simulink model "SRS_MBC_Ioniq5_17_Carsim_ACC_final"  (R2023b)
settings: Solver=FixedStepAuto  StartTime=0.0  StopTime=200  FixedStep=0.001  MaxStep=0.001  RelTol=1e-3
libraries: slpidlib x3, Solver_SF x1
settings Model: DataTypeOverride=Double  MinMaxOverflowLogging=ForceOff  PacingRate=1.100000  Creator=황수빈  LastModifiedBy=황수빈

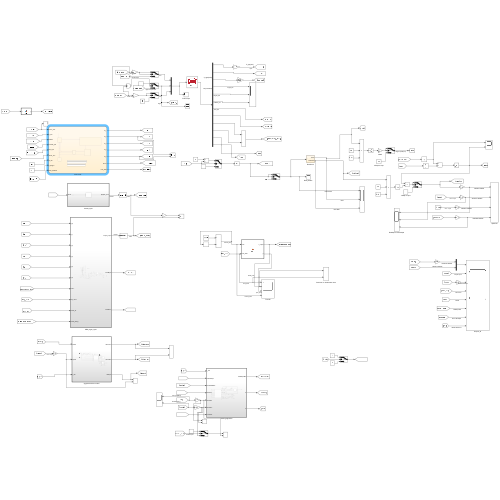
[thumbnail: Simulink's stored preview of the top-level diagram]
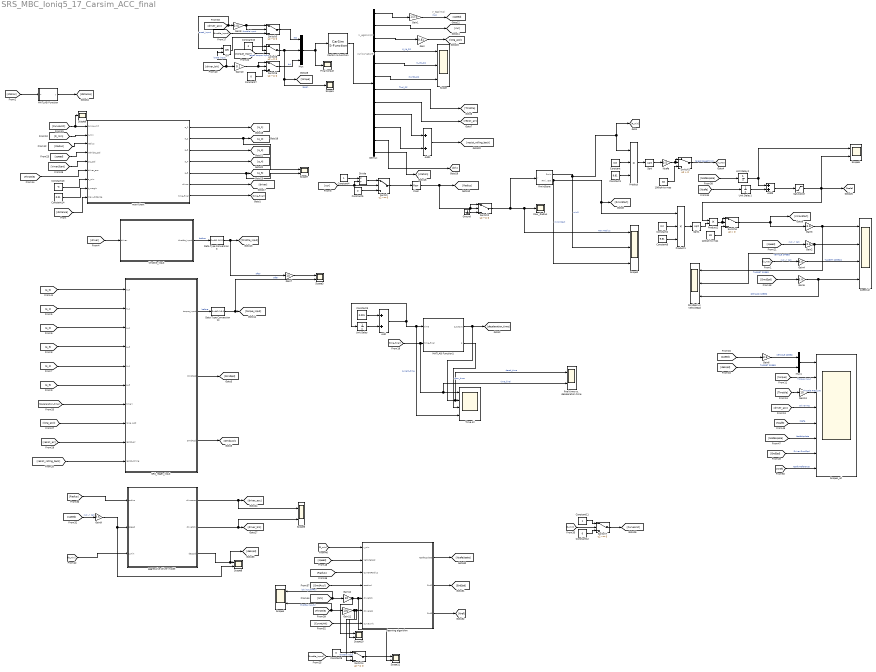
== system SRS_MBC_Ioniq5_17_Carsim_ACC_final ==
  note: V_ego(km/h)
  note: V_ego(m/s)
  note: cur(curvature)
  100kph to mps : Constant  Value=33
  120kph to mps : Constant  Value=33
  Add : Sum
  Add1 : Sum
  Add3 : Sum
  CarSim S-Function : Solver_SF/CarSim S-Function  Priority=1  SIMFILE=simfile.sim  Run_RTs=off  vs_state_ind=Run  StopMode_ind=Vehicle Model
  Constant : Constant  Value=0.8
  Constant1 : Constant  Value=9.81
  Constant{5,7..8,10,12} (5 alike) : Constant  Value=0
  Constant11 : Constant
  Constant13 : Constant  Value=-3
  Constant14 : Constant  Value=0.01
  Constant2 : Constant  Value=0.2
  Constant3 : Constant  Value=0.001
  Constant4 : Constant
  Constant6 : Constant  Value=9.81
  Data Type Conversion14 : DataTypeConversion  OutDataTypeStr=fixdt(1,16,0)  RndMeth=Nearest  SaturateOnIntegerOverflow=off
  Data Type Conversion3 : DataTypeConversion  OutDataTypeStr=fixdt(1,16,0)  RndMeth=Nearest  SaturateOnIntegerOverflow=off
  Demux : Demux  Outputs=12
  Divide : Product  Inputs=*/
  DmdSpd vs VehicleSpd : Scope  NumInputPorts=3
  Final torque : Scope
  Floor : Rounding
  Gain : Gain  Gain=9.81
  Gain1 : Gain  Gain=1/3.6
  Gain10 : Gain  Gain=0.1
  Gain11 : Gain  Gain=100
  Gain12 : Gain  Gain=10
  Gain13 : Gain  Gain=10
  Gain{2..6,9} (6 alike) : Gain  Gain=3.6
  Gain7 : Gain  Gain=10
  Gain8 : Gain  Gain=0.01
  Ground : Ground
  MATLAB Function : MATLAB Function  TreatAsAtomicUnit=on
  MATLAB Function1 : MATLAB Function  TreatAsAtomicUnit=on
  Mux : Mux  Inputs=3
  Mux1 : Mux  Inputs=2
  Nsafe : Gain  Gain=0.5
  OR : Logic  Operator=OR  IconShape=distinctive  AllPortsSameDT=off  OutDataTypeStr=boolean
  Product : Product  Inputs=3
  Product1 : Product  Inputs=3
  Product2 : Product
  Raw_Radius : Scope
  RminStore : Stateflow chart  TreatAsAtomicUnit=on
  SRS_regen_input : Subsystem  TreatAsAtomicUnit=on
  Saturation : Saturate  UpperLimit=1.2  LowerLimit=0.8
  Scope : Scope  NumInputPorts=3
  Scope1 : Scope
  Scope{3..8,10..11} (8 alike) : Scope  NumInputPorts=2
  Scope2 : Scope  NumInputPorts=3
  Scope9 : Scope
  Scopes_all : Scope  NumInputPorts=8
  Sqrt : Sqrt
  Sqrt1 : Sqrt
  Switch{,2,4..8} (7 alike) : Switch  Criteria=u2 ~= 0  SaturateOnIntegerOverflow=off  InputSameDT=off
  Switch1 : Switch  Criteria=u2 > Threshold  SaturateOnIntegerOverflow=off  InputSameDT=off
  Switch3 : Switch  Criteria=u2 > Threshold  SaturateOnIntegerOverflow=off  InputSameDT=off
  Time All : Scope  NumInputPorts=4
  Unit Delay : UnitDelay  SampleTime=-1  HasFrameUpgradeWarning=on
  Unit Delay1 : UnitDelay  InitialCondition=1  SampleTime=-1  HasFrameUpgradeWarning=on
  Unit Delay2 : UnitDelay  SampleTime=-1  HasFrameUpgradeWarning=on
  aggressive driver model : Subsystem  TreatAsAtomicUnit=on
  final time vs. deceleration time : Scope  NumInputPorts=2
  learning algorithm : Subsystem  TreatAsAtomicUnit=on
  main chart : Stateflow chart  TreatAsAtomicUnit=on
  speed all : Scope  NumInputPorts=4
  throttle_input : Subsystem  TreatAsAtomicUnit=on  SystemSampleTime=0.01
  wires:
  Switch/1 -> Floor/1
  [cur] -> Switch/2, Divide/2
  Constant5/1 -> Switch/3
  Constant4/1 -> Divide/1
  Divide/1 -> Switch/1
  Demux/1 -> Gain1/1
  Demux/2 -> [cur]
  Gain1/1 -> [speed]  "mps"
  CarSim S-Function/1 -> Demux/1
  [driver] -> throttle_input/1(driver)
  Data Type Conversion3/1 -> Gain7/1, [throttle_input]  "after"
  throttle_input/1(throttle_input) -> Data Type Conversion3/1  "before"
  SRS_regen_input/1(torque_input) -> Data Type Conversion14/1  "before"
  [a_2] -> SRS_regen_input/3(a_2)
  Data Type Conversion14/1 -> Scope3/2, [torque_input]  "after"
  [a_0] -> SRS_regen_input/1(a_0)
  [a_3] -> SRS_regen_input/4(a_3)
  [a_5] -> SRS_regen_input/6(a_5)
  Demux/3 -> Gain/1
  [a_1] -> SRS_regen_input/2(a_1)
  [a_4] -> SRS_regen_input/5(a_4)
  [speed] -> main chart/4(vehicle_spd)
  [VmaxStart] -> main chart/5(srs_spd)
  main chart/2(a_2) -> Scope7/1, [a_2]
  main chart/3(a_3) -> [a_3]
  main chart/4(a_4) -> [a_4]
  main chart/1(a_1) -> [a_1]
  main chart/5(a_5) -> Scope7/2, [a_5]
  main chart/6(driver) -> [driver]
  [V_max] -> Gain4/1  "m/s -> kph"
  [R_min] -> main chart/2(r_min)
  main chart/7(time_final) -> [time_final]
  Add/1 -> Unit Delay/1, Time All/4, MATLAB Function1/1(time)  "current_time"
  Gain2/1 -> DmdSpd vs VehicleSpd/2, speed all/2  "VEHICLE SPEED"
  [speed] -> Gain2/1  "m/s -> kph"
  [time_final] -> final time vs. deceleration time/2, Time All/1, MATLAB Function1/2(time_final)  "time_final"
  [Radius] -> main chart/3(radius)
  Mux/1 -> Final torque/1, CarSim S-Function/1
  Constant3/1 -> Add/1
  Unit Delay/1 -> Add/2
  MATLAB Function1/1(t_output) -> final time vs. deceleration time/1, Time All/2, [deceleration_time]  "decel_time"
  Constant1/1 -> Product/3
  100kph to mps/1 -> Switch1/3
  Product/1 -> Sqrt/1
  Constant/1 -> Product/2
  Sqrt/1 -> Nsafe/1
  Nsafe/1 -> Switch1/1, Switch1/2
  Switch2/1 -> Scope2/1, Raw_Radius/1, RminStore/1(r)  "Raw Radius"
  Switch1/1 -> [V_max]  "target speed(m/s)"
  Floor/1 -> Switch2/1, Switch2/2, [Radius]
  Ground/1 -> Switch2/3
  MATLAB Function1/2(p) -> Time All/3  "prev_time"
  [deceleration_time] -> SRS_regen_input/7(time t)
  [long_accl] -> SRS_regen_input/8(long. accl)
  Product2/1 -> Switch3/1, Switch3/2
  120kph to mps/1 -> Switch3/3
  Constant6/1 -> Product1/3
  Sqrt1/1 -> Product2/2
  Constant2/1 -> Product1/2
  Product1/1 -> Sqrt1/1
  RminStore/1(Rmin) -> Product/1, [R_min], Scope2/2  "minR"
  Switch3/1 -> Gain3/1, [VmaxStart]
  Gain3/1 -> DmdSpd vs VehicleSpd/1, speed all/1  "TARGET SPEED"
  SRS_regen_input/2(DmdSpd) -> [DmdSpd]
  [DmdSpd] -> Gain5/1
  Gain5/1 -> DmdSpd vs VehicleSpd/3, speed all/4  "DEMAND SPEED"
  Gain4/1 -> speed all/3  "TARGET SPEED2"
  RminStore/2(RminStart) -> Scope2/3, [RminStart], Product1/1  "minR Start"
  Demux/4 -> Scope/1  "M_Mt_D2"
  Demux/5 -> Scope/2  "M_Mtr_D2"
  Demux/6 -> Scope/3  "PwMtC_D2"
  Demux/7 -> [Throttle]  "Thrtl_SC"
  SRS_regen_input/3(DmdAccl) -> [DmdAccl]
  [speed] -> Gain6/1
  [desspd] -> Mux1/2  "TARGET SPEED"
  Gain6/1 -> Mux1/1  "VEHICLE SPEED"
  Mux1/1 -> Scopes_all/1
  [Throttle] -> Gain13/1
  Demux/8 -> [resist_air]
  Demux/9 -> Add1/1
  Demux/10 -> Add1/2
  Add1/1 -> [resist_rolling_back]
  [resist_air] -> SRS_regen_input/9(resist_air)
  [resist_rolling_back] -> SRS_regen_input/10(resist_rolling)
  aggressive driver model/1(driveracc) -> Scope5/1, [driver_acc]
  [Radius] -> aggressive driver model/1(radius)
  Gain9/1 -> Scope8/2, aggressive driver model/2(speed)
  [speed] -> Gain9/1  "m/s -> kph"
  [throttle_input] -> Switch5/3  "throttle input"
  [Nsafe] -> Unit Delay1/1
  aggressive driver model/2(driverbrk) -> Scope5/2, [driver_brk]
  [driver_brk] -> OR/2, Gain10/1  "brake input"
  [speed] -> learning algorithm/2(VehicleSpd)
  [DmdAccl] -> learning algorithm/4(accdmd)
  [CurveUnit] -> learning algorithm/7(curveunit)
  [R_min] -> learning algorithm/1(r_min)
  learning algorithm/1(NsafeUpdate) -> [NsafeUpate]
  Switch7/1 -> [CurveUnit]
  Constant11/1 -> Switch7/1
  [R_min] -> Switch7/2
  Constant12/1 -> Switch7/3
  [Radius] -> learning algorithm/3(CurrentRadius)
  Demux/11 -> [brk]
  Unit Delay1/1 -> Add3/2
  Saturation/1 -> Product2/1, [Nsafe], Scope6/2
  Add3/1 -> Saturation/1
  [NsafeUpate] -> Unit Delay2/1
  Unit Delay2/1 -> Scope6/1, Add3/1
  [R_min] -> aggressive driver model/3(r_min)
  aggressive driver model/3(desspd) -> [desspd], Scope8/1
  [driver_acc] -> OR/1, Gain8/1  "accel_input"
  Switch8/1 -> Mux/2, Scope1/1, [torque]  "regen"
  Constant7/1 -> Switch6/3
  [torque_input] -> Switch8/3  "regen torque input"
  Constant10/1 -> Switch8/1
  Gain8/1 -> Switch5/2, Switch5/1
  [CurveUnit] -> Scope9/1, main chart/1(curve_unit)
  [torque] -> Scopes_all/2  "Torque Input"
  [driver_acc] -> Scopes_all/4  "Driver Acc"
  [Nsafe] -> Scopes_all/5  "Nsafe"
  learning algorithm/2(Out2) -> [EndSpd]
  learning algorithm/3(Out3) -> [Nref]
  [NsafeUpate] -> Scopes_all/6  "NsafeUpdate"
  [EndSpd] -> Scopes_all/7  "Driver DmdSpd"
  [Nref] -> Scopes_all/8  "Nsafe Reference"
  Constant13/1 -> main chart/7(a_min)
  Constant14/1 -> main chart/8(t_margin)
  MATLAB Function/1(y) -> [distance]
  [station] -> MATLAB Function/1(u)
  [distance] -> main chart/9(max_distance)
  Gain/1 -> [long_accl]
  Gain7/1 -> Scope3/1
  Demux/12 -> [station]
  [Throttle] -> main chart/6(driver_acc)
  [brk] -> Gain12/1, Scope4/1  "brk input(MPa)"
  [Throttle] -> Gain11/1, Scope4/2  "throttle input(-)"
  Gain13/1 -> Scopes_all/3  "Throttle Pressure"
  Gain11/1 -> Switch4/3, Scope10/2, learning algorithm/6(driveracc)
  Switch5/1 -> Mux/1  "acc"
  Gain10/1 -> Switch6/1, Switch6/2
  OR/1 -> Switch8/2
  Switch6/1 -> Mux/3  "brk"
  Gain12/1 -> Scope10/1, Scope11/2, learning algorithm/5(drvierbrk)
  [throttle_input] -> Switch4/2  "throttle input"
  Switch4/1 -> Scope11/1
  Constant8/1 -> Switch4/1

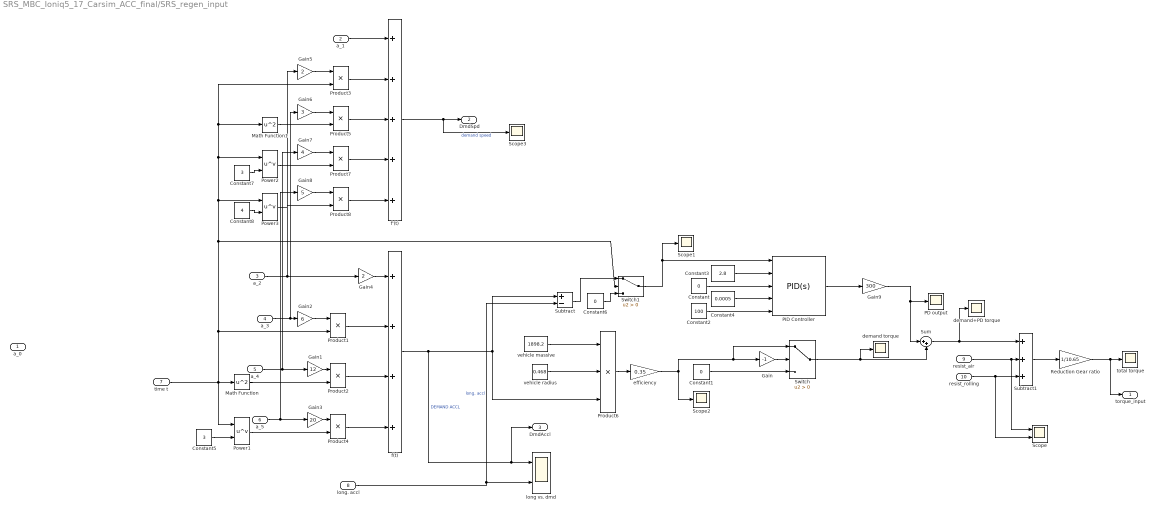
== system SRS_MBC_Ioniq5_17_Carsim_ACC_final/SRS_regen_input ==
  a_0 : Inport
  a_1 : Inport  Port=2
  a_2 : Inport  Port=3
  a_3 : Inport  Port=4
  a_4 : Inport  Port=5
  a_5 : Inport  Port=6
  time t : Inport  Port=7
  long. accl : Inport  Port=8
  resist_air : Inport  Port=9
  resist_rolling : Inport  Port=10
  Constant : Constant  Value=0
  Constant1 : Constant  Value=0
  Constant2 : Constant  Value=100
  Constant3 : Constant  Value=2.8
  Constant4 : Constant  Value=0.0005
  Constant5 : Constant  Value=3
  Constant6 : Constant  Value=0
  Constant7 : Constant  Value=3
  Constant8 : Constant  Value=4
  Gain : Gain  Gain=-1
  Gain1 : Gain  Gain=12
  Gain2 : Gain  Gain=6
  Gain3 : Gain  Gain=20
  Gain4 : Gain  Gain=2
  Gain5 : Gain  Gain=2
  Gain6 : Gain  Gain=3
  Gain7 : Gain  Gain=4
  Gain8 : Gain  Gain=5
  Gain9 : Gain  Gain=300
  Math Function : Math  Operator=square
  Math Function1 : Math  Operator=square
  PD output : Scope
  PID Controller : slpidlib/PID Controller  Controller=PID  Form=Parallel  TimeDomain=Continuous-time  UseExternalTs=off  SampleTime=-1  IntegratorMethod=Forward Euler  FilterMethod=Forward Euler  ControllerParametersSource=external  P=1  I=1  UseKiTs=off  D=0  N=100  UseFilter=on  TunerSelectOption=Transfer Function Based (PID Tuner App)  InitialConditionSource=internal  InitialConditionForIntegrator=0  InitialConditionForFilter=0  DifferentiatorICPrevScaledInput=0  ExternalReset=none  TrackingMode=off  Kt=1  LimitOutput=off  SatLimitsSource=internal  UpperSaturationLimit=inf  LowerSaturationLimit=-inf  LinearizeAsGain=on  AntiWindupMode=none  Kb=1  LimitIntegrator=off  UpperIntegratorSaturationLimit=inf  LowerIntegratorSaturationLimit=-inf  POutMin=[]  POutMax=[]  IOutMin=[]  IOutMax=[]  DOutMin=[]  DOutMax=[]  NOutMin=[]  NOutMax=[]  SumOutMin=[]  SumOutMax=[]  SaturationOutMin=[]  SaturationOutMax=[]  PParamMin=[]  PParamMax=[]  IParamMin=[]  IParamMax=[]  DParamMin=[]  DParamMax=[]  NParamMin=[]  NParamMax=[]  KbParamMin=[]  KbParamMax=[]  KtParamMin=[]  KtParamMax=[]  KbOutMin=[]  KbOutMax=[]  KtOutMin=[]  KtOutMax=[]  IntegratorOutMin=[]  IntegratorOutMax=[]  FilterOutMin=[]  FilterOutMax=[]  SumI1OutMin=[]  SumI1OutMax=[]  SumI2OutMin=[]  SumI2OutMax=[]  SumI3OutMin=[]  SumI3OutMax=[]  SumI4OutMin=[]  SumI4OutMax=[]  SumDOutMin=[]  SumDOutMax=[]  DifferentiatorOutMin=[]  DifferentiatorOutMax=[]  FilterDiffOutCoefMin=[]  FilterDiffOutCoefMax=[]  ReciprocalOutMin=[]  ReciprocalOutMax=[]  SumDenOutMin=[]  SumDenOutMax=[]  SumNumOutMin=[]  SumNumOutMax=[]  DivideOutMin=[]  DivideOutMax=[]  UdiffTsProdOutMin=[]  UdiffTsProdOutMax=[]  NTsProdOutMin=[]  NTsProdOutMax=[]  UintegralTsProdOutMin=[]  UintegralTsProdOutMax=[]  UngainTsProdOutMin=[]  UngainTsProdOutMax=[]  ClampingZeroOutDataTypeStr=Inherit: Inherit via back propagation  ClampingZeroOutMin=[]  ClampingZeroOutMax=[]  FilterDenConstantOutDataTypeStr=Inherit: Inherit via back propagation  FilterDenConstantOutMin=[]  FilterDenConstantOutMax=[]  PCopyOutDataTypeStr=Inherit: Inherit via back propagation  PCopyOutMin=[]  PCopyOutMax=[]  NCopyOutDataTypeStr=Inherit: Inherit via back propagation  NCopyOutMin=[]  NCopyOutMax=[]  IntegratorContinuousStateAttributes=''  IntegratorStateMustResolveToSignalObject=off  IntegratorRTWStateStorageClass=Auto  FilterContinuousStateAttributes=''  FilterStateMustResolveToSignalObject=off  FilterRTWStateStorageClass=Auto  ParallelPVariant=ExternalParameters  IdealPVariant=Disabled  IVariant=ExternalParameters  DVariant=ExternalParameters  IntegratorVariant=Continuous  SatVariant=Disabled  AWVariant=Passthrough  PCopyVariant=Disabled  TRVariant=Disabled  FdbkBlocksVariant=Forward  IdealPFdbkVariant=Disabled  SatFdbkVariant=Disabled  DerivativeFilterVariant=ContFilter  NVariant=ExternalParameters  NCopyVariant=Disabled  FilterICVariant=InternalICsFilter  IntegratorICVariant=InternalICs  ExternalResetVariant=Disabled  TRSumVariant=Passthrough  SumFdbkVariant=Disabled  SumVariant=Sum_PID  TsampFilterVariant=InternalTs  TsampNgainVariant=Passthrough  TsampIntegralVariant=Disabled_SignalSpec  ExternalSaturationOutDataTypeStr=Inherit: Same as second input
  Power1 : Math  Operator=pow
  Power2 : Math  Operator=pow
  Power3 : Math  Operator=pow
  Product{1..5,7..8} (7 alike) : Product
  Product6 : Product  Inputs=3
  Reduction Gear ratio : Gain  Gain=1/10.65
  Scope : Scope  NumInputPorts=2
  Scope1 : Scope
  Scope2 : Scope
  Scope3 : Scope
  Subtract : Sum  Inputs=+-
  Subtract1 : Sum  Inputs=+++
  Sum : Sum  Inputs=|++
  Switch : Switch  Criteria=u2 > Threshold  SaturateOnIntegerOverflow=off  InputSameDT=off
  Switch1 : Switch  Criteria=u2 > Threshold  SaturateOnIntegerOverflow=off  InputSameDT=off
  demand torque : Scope
  demand+PD torque : Scope
  efficiency : Gain  Gain=0.35
  f'(t) : Sum  Inputs=5
  f(t) : Sum  Inputs=4
  long vs. dmd : Scope  NumInputPorts=2
  total torque : Scope
  vehicle massive : Constant  Value=1898.2
  vehicle radius : Constant  Value=0.468
  torque_input : Outport
  DmdSpd : Outport  Port=2
  DmdAccl : Outport  Port=3
  wires:
  time t/1 -> Power3/1, Power2/1, Math Function1/1, Product3/2, Switch1/2, Product1/2, Power1/1, Math Function/1
  Constant5/1 -> Power1/2
  Product2/1 -> f(t)/3
  Product4/1 -> f(t)/4
  Power1/1 -> Product4/2
  Math Function/1 -> Product2/2
  Product6/1 -> efficiency/1
  efficiency/1 -> Scope2/1, Switch/1, Gain/1
  Constant1/1 -> Switch/3
  Gain/1 -> Switch/2
  f(t)/1 -> Product6/3, Subtract/1, DmdAccl/1, long vs. dmd/1  "DEMAND ACCL"
  a_2/1 -> Gain4/1, Gain5/1
  a_4/1 -> Gain1/1, Gain7/1
  Gain1/1 -> Product2/1
  a_5/1 -> Gain8/1, Gain3/1
  Gain3/1 -> Product4/1
  Gain4/1 -> f(t)/1
  a_3/1 -> Gain6/1, Gain2/1
  Gain2/1 -> Product1/1
  Product1/1 -> f(t)/2
  long. accl/1 -> Subtract/2, long vs. dmd/2  "long. accl"
  Subtract/1 -> Switch1/1
  Switch1/1 -> PID Controller/1, Scope1/1
  Constant6/1 -> Switch1/3
  Constant2/1 -> PID Controller/5
  Constant4/1 -> PID Controller/4
  Constant/1 -> PID Controller/3
  Constant3/1 -> PID Controller/2
  PID Controller/1 -> Gain9/1
  a_1/1 -> f'(t)/1
  Product3/1 -> f'(t)/2
  Product5/1 -> f'(t)/3
  Product7/1 -> f'(t)/4
  Product8/1 -> f'(t)/5
  Gain5/1 -> Product3/1
  Gain6/1 -> Product5/1
  Gain7/1 -> Product7/1
  Gain8/1 -> Product8/1
  f'(t)/1 -> Scope3/1, DmdSpd/1  "demand speed"
  Math Function1/1 -> Product5/2
  Power2/1 -> Product7/2
  Power3/1 -> Product8/2
  Constant7/1 -> Power2/2
  Constant8/1 -> Power3/2
  Switch/1 -> Sum/2, demand torque/1
  vehicle radius/1 -> Product6/2
  vehicle massive/1 -> Product6/1
  Sum/1 -> demand+PD torque/1, Subtract1/1
  Gain9/1 -> PD output/1, Sum/1
  Reduction Gear ratio/1 -> torque_input/1, total torque/1
  resist_rolling/1 -> Scope/2, Subtract1/3
  resist_air/1 -> Scope/1, Subtract1/2
  Subtract1/1 -> Reduction Gear ratio/1

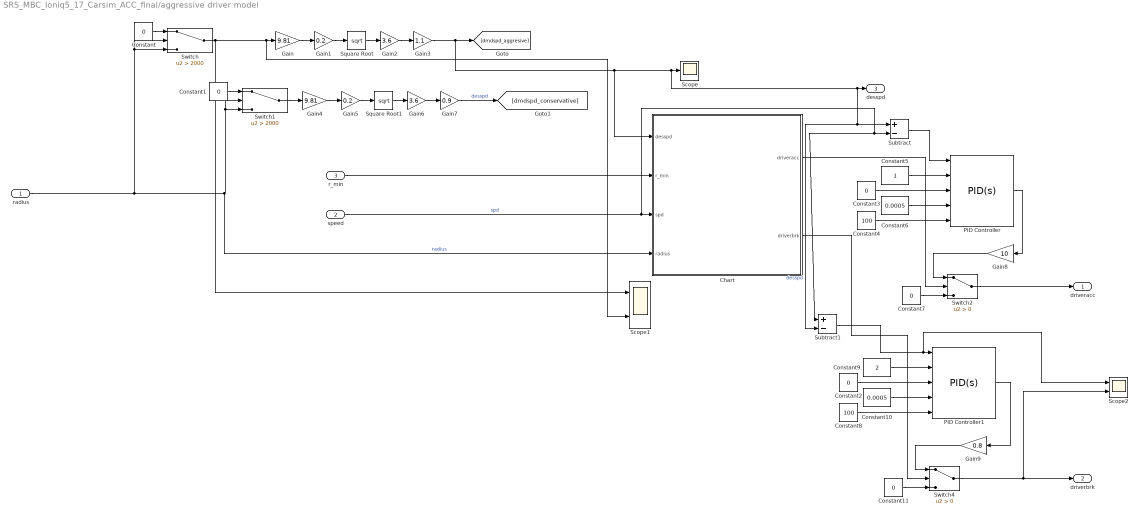
== system SRS_MBC_Ioniq5_17_Carsim_ACC_final/aggressive driver model ==
  radius : Inport
  speed : Inport  Port=2
  r_min : Inport  Port=3
  Chart : Stateflow chart  TreatAsAtomicUnit=on
  Constant{,1..3,7,11} (6 alike) : Constant  Value=0
  Constant10 : Constant  Value=0.0005
  Constant4 : Constant  Value=100
  Constant5 : Constant
  Constant6 : Constant  Value=0.0005
  Constant8 : Constant  Value=100
  Constant9 : Constant  Value=2
  Gain : Gain  Gain=9.81
  Gain1 : Gain  Gain=0.2
  Gain2 : Gain  Gain=3.6
  Gain3 : Gain  Gain=1.1
  Gain4 : Gain  Gain=9.81
  Gain5 : Gain  Gain=0.2
  Gain6 : Gain  Gain=3.6
  Gain7 : Gain  Gain=0.9
  Gain8 : Gain  Gain=10
  Gain9 : Gain  Gain=0.8
  PID Controller : slpidlib/PID Controller  Controller=PID  Form=Parallel  TimeDomain=Continuous-time  UseExternalTs=off  SampleTime=-1  IntegratorMethod=Forward Euler  FilterMethod=Forward Euler  ControllerParametersSource=external  P=1  I=1  UseKiTs=off  D=0  N=100  UseFilter=on  TunerSelectOption=Transfer Function Based (PID Tuner App)  InitialConditionSource=internal  InitialConditionForIntegrator=0  InitialConditionForFilter=0  DifferentiatorICPrevScaledInput=0  ExternalReset=none  TrackingMode=off  Kt=1  LimitOutput=off  SatLimitsSource=internal  UpperSaturationLimit=inf  LowerSaturationLimit=-inf  LinearizeAsGain=on  AntiWindupMode=none  Kb=1  LimitIntegrator=off  UpperIntegratorSaturationLimit=inf  LowerIntegratorSaturationLimit=-inf  POutMin=[]  POutMax=[]  IOutMin=[]  IOutMax=[]  DOutMin=[]  DOutMax=[]  NOutMin=[]  NOutMax=[]  SumOutMin=[]  SumOutMax=[]  SaturationOutMin=[]  SaturationOutMax=[]  PParamMin=[]  PParamMax=[]  IParamMin=[]  IParamMax=[]  DParamMin=[]  DParamMax=[]  NParamMin=[]  NParamMax=[]  KbParamMin=[]  KbParamMax=[]  KtParamMin=[]  KtParamMax=[]  KbOutMin=[]  KbOutMax=[]  KtOutMin=[]  KtOutMax=[]  IntegratorOutMin=[]  IntegratorOutMax=[]  FilterOutMin=[]  FilterOutMax=[]  SumI1OutMin=[]  SumI1OutMax=[]  SumI2OutMin=[]  SumI2OutMax=[]  SumI3OutMin=[]  SumI3OutMax=[]  SumI4OutMin=[]  SumI4OutMax=[]  SumDOutMin=[]  SumDOutMax=[]  DifferentiatorOutMin=[]  DifferentiatorOutMax=[]  FilterDiffOutCoefMin=[]  FilterDiffOutCoefMax=[]  ReciprocalOutMin=[]  ReciprocalOutMax=[]  SumDenOutMin=[]  SumDenOutMax=[]  SumNumOutMin=[]  SumNumOutMax=[]  DivideOutMin=[]  DivideOutMax=[]  UdiffTsProdOutMin=[]  UdiffTsProdOutMax=[]  NTsProdOutMin=[]  NTsProdOutMax=[]  UintegralTsProdOutMin=[]  UintegralTsProdOutMax=[]  UngainTsProdOutMin=[]  UngainTsProdOutMax=[]  ClampingZeroOutDataTypeStr=Inherit: Inherit via back propagation  ClampingZeroOutMin=[]  ClampingZeroOutMax=[]  FilterDenConstantOutDataTypeStr=Inherit: Inherit via back propagation  FilterDenConstantOutMin=[]  FilterDenConstantOutMax=[]  PCopyOutDataTypeStr=Inherit: Inherit via back propagation  PCopyOutMin=[]  PCopyOutMax=[]  NCopyOutDataTypeStr=Inherit: Inherit via back propagation  NCopyOutMin=[]  NCopyOutMax=[]  IntegratorContinuousStateAttributes=''  IntegratorStateMustResolveToSignalObject=off  IntegratorRTWStateStorageClass=Auto  FilterContinuousStateAttributes=''  FilterStateMustResolveToSignalObject=off  FilterRTWStateStorageClass=Auto  ParallelPVariant=ExternalParameters  IdealPVariant=Disabled  IVariant=ExternalParameters  DVariant=ExternalParameters  IntegratorVariant=Continuous  SatVariant=Disabled  AWVariant=Passthrough  PCopyVariant=Disabled  TRVariant=Disabled  FdbkBlocksVariant=Forward  IdealPFdbkVariant=Disabled  SatFdbkVariant=Disabled  DerivativeFilterVariant=ContFilter  NVariant=ExternalParameters  NCopyVariant=Disabled  FilterICVariant=InternalICsFilter  IntegratorICVariant=InternalICs  ExternalResetVariant=Disabled  TRSumVariant=Passthrough  SumFdbkVariant=Disabled  SumVariant=Sum_PID  TsampFilterVariant=InternalTs  TsampNgainVariant=Passthrough  TsampIntegralVariant=Disabled_SignalSpec  ExternalSaturationOutDataTypeStr=Inherit: Same as second input
  PID Controller1 : slpidlib/PID Controller  Controller=PID  Form=Parallel  TimeDomain=Continuous-time  UseExternalTs=off  SampleTime=-1  IntegratorMethod=Forward Euler  FilterMethod=Forward Euler  ControllerParametersSource=external  P=1  I=1  UseKiTs=off  D=0  N=100  UseFilter=on  TunerSelectOption=Transfer Function Based (PID Tuner App)  InitialConditionSource=internal  InitialConditionForIntegrator=0  InitialConditionForFilter=0  DifferentiatorICPrevScaledInput=0  ExternalReset=none  TrackingMode=off  Kt=1  LimitOutput=off  SatLimitsSource=internal  UpperSaturationLimit=inf  LowerSaturationLimit=-inf  LinearizeAsGain=on  AntiWindupMode=none  Kb=1  LimitIntegrator=off  UpperIntegratorSaturationLimit=inf  LowerIntegratorSaturationLimit=-inf  POutMin=[]  POutMax=[]  IOutMin=[]  IOutMax=[]  DOutMin=[]  DOutMax=[]  NOutMin=[]  NOutMax=[]  SumOutMin=[]  SumOutMax=[]  SaturationOutMin=[]  SaturationOutMax=[]  PParamMin=[]  PParamMax=[]  IParamMin=[]  IParamMax=[]  DParamMin=[]  DParamMax=[]  NParamMin=[]  NParamMax=[]  KbParamMin=[]  KbParamMax=[]  KtParamMin=[]  KtParamMax=[]  KbOutMin=[]  KbOutMax=[]  KtOutMin=[]  KtOutMax=[]  IntegratorOutMin=[]  IntegratorOutMax=[]  FilterOutMin=[]  FilterOutMax=[]  SumI1OutMin=[]  SumI1OutMax=[]  SumI2OutMin=[]  SumI2OutMax=[]  SumI3OutMin=[]  SumI3OutMax=[]  SumI4OutMin=[]  SumI4OutMax=[]  SumDOutMin=[]  SumDOutMax=[]  DifferentiatorOutMin=[]  DifferentiatorOutMax=[]  FilterDiffOutCoefMin=[]  FilterDiffOutCoefMax=[]  ReciprocalOutMin=[]  ReciprocalOutMax=[]  SumDenOutMin=[]  SumDenOutMax=[]  SumNumOutMin=[]  SumNumOutMax=[]  DivideOutMin=[]  DivideOutMax=[]  UdiffTsProdOutMin=[]  UdiffTsProdOutMax=[]  NTsProdOutMin=[]  NTsProdOutMax=[]  UintegralTsProdOutMin=[]  UintegralTsProdOutMax=[]  UngainTsProdOutMin=[]  UngainTsProdOutMax=[]  ClampingZeroOutDataTypeStr=Inherit: Inherit via back propagation  ClampingZeroOutMin=[]  ClampingZeroOutMax=[]  FilterDenConstantOutDataTypeStr=Inherit: Inherit via back propagation  FilterDenConstantOutMin=[]  FilterDenConstantOutMax=[]  PCopyOutDataTypeStr=Inherit: Inherit via back propagation  PCopyOutMin=[]  PCopyOutMax=[]  NCopyOutDataTypeStr=Inherit: Inherit via back propagation  NCopyOutMin=[]  NCopyOutMax=[]  IntegratorContinuousStateAttributes=''  IntegratorStateMustResolveToSignalObject=off  IntegratorRTWStateStorageClass=Auto  FilterContinuousStateAttributes=''  FilterStateMustResolveToSignalObject=off  FilterRTWStateStorageClass=Auto  ParallelPVariant=ExternalParameters  IdealPVariant=Disabled  IVariant=ExternalParameters  DVariant=ExternalParameters  IntegratorVariant=Continuous  SatVariant=Disabled  AWVariant=Passthrough  PCopyVariant=Disabled  TRVariant=Disabled  FdbkBlocksVariant=Forward  IdealPFdbkVariant=Disabled  SatFdbkVariant=Disabled  DerivativeFilterVariant=ContFilter  NVariant=ExternalParameters  NCopyVariant=Disabled  FilterICVariant=InternalICsFilter  IntegratorICVariant=InternalICs  ExternalResetVariant=Disabled  TRSumVariant=Passthrough  SumFdbkVariant=Disabled  SumVariant=Sum_PID  TsampFilterVariant=InternalTs  TsampNgainVariant=Passthrough  TsampIntegralVariant=Disabled_SignalSpec  ExternalSaturationOutDataTypeStr=Inherit: Same as second input
  Scope : Scope
  Scope1 : Scope  NumInputPorts=2
  Scope2 : Scope  NumInputPorts=2
  Square Root : Sqrt
  Square Root1 : Sqrt
  Subtract : Sum  Inputs=+-
  Subtract1 : Sum  Inputs=+-
  Switch : Switch  Criteria=u2 > Threshold  Threshold=2000  SaturateOnIntegerOverflow=off  InputSameDT=off
  Switch1 : Switch  Criteria=u2 > Threshold  Threshold=2000  SaturateOnIntegerOverflow=off  InputSameDT=off
  Switch2 : Switch  Criteria=u2 > Threshold  SaturateOnIntegerOverflow=off  InputSameDT=off
  Switch4 : Switch  Criteria=u2 > Threshold  SaturateOnIntegerOverflow=off  InputSameDT=off
  driveracc : Outport
  driverbrk : Outport  Port=2
  desspd : Outport  Port=3
  wires:
  radius/1 -> Chart/4(radius), Switch1/2, Switch1/3, Switch/2, Switch/3  "radius"
  speed/1 -> Subtract1/1, Subtract/2, Chart/3(spd)  "spd"
  Gain/1 -> Gain1/1
  Gain1/1 -> Square Root/1
  Square Root/1 -> Gain2/1
  Gain2/1 -> Gain3/1
  Constant/1 -> Switch/1
  Switch1/1 -> Gain4/1
  Constant1/1 -> Switch1/1
  Square Root1/1 -> Gain6/1
  Gain5/1 -> Square Root1/1
  Gain6/1 -> Gain7/1
  Gain4/1 -> Gain5/1
  Gain3/1 -> Chart/1(desspd), Subtract1/2, Subtract/1, desspd/1, Scope/1, [dmdspd_aggresive]  "desspd"
  Gain7/1 -> [dmdspd_conservative]  "desspd"
  r_min/1 -> Chart/2(r_min)
  Subtract/1 -> PID Controller/1
  Constant4/1 -> PID Controller/5
  Constant6/1 -> PID Controller/4
  Constant3/1 -> PID Controller/3
  Constant5/1 -> PID Controller/2
  PID Controller/1 -> Gain8/1
  Constant7/1 -> Switch2/3
  Chart/1(driveracc) -> Switch2/2
  Switch2/1 -> driveracc/1
  Switch/1 -> Scope1/2, Gain/1, Scope1/1
  Constant11/1 -> Switch4/3
  Subtract1/1 -> Scope2/1, PID Controller1/1
  PID Controller1/1 -> Gain9/1
  Constant9/1 -> PID Controller1/2
  Constant10/1 -> PID Controller1/4
  Constant2/1 -> PID Controller1/3
  Constant8/1 -> PID Controller1/5
  Chart/2(driverbrk) -> Switch4/2
  Switch4/1 -> Scope2/2, driverbrk/1
  Gain8/1 -> Switch2/1
  Gain9/1 -> Switch4/1

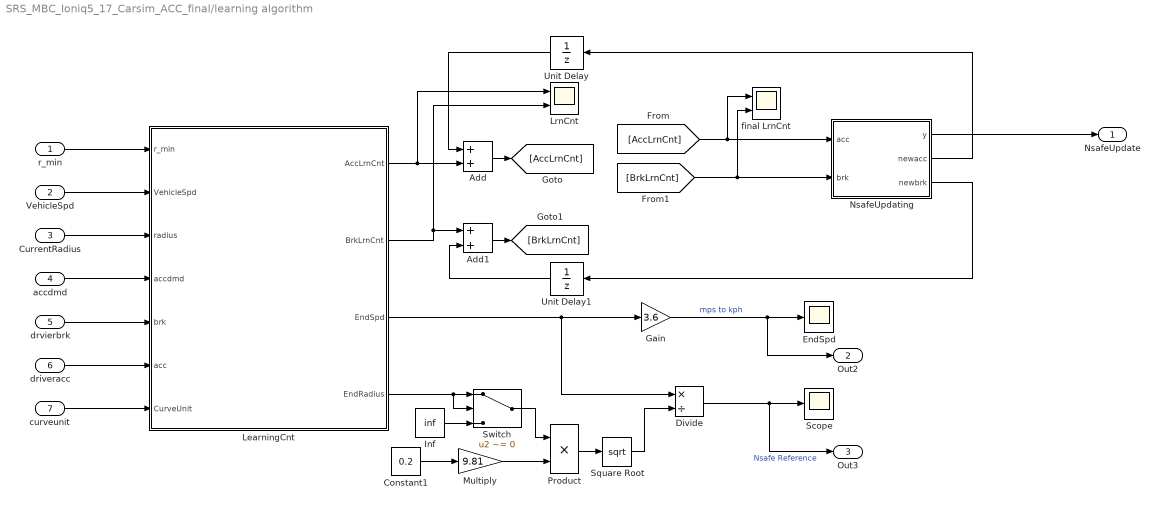
== system SRS_MBC_Ioniq5_17_Carsim_ACC_final/learning algorithm ==
  r_min : Inport
  VehicleSpd : Inport  Port=2
  CurrentRadius : Inport  Port=3
  accdmd : Inport  Port=4
  drvierbrk : Inport  Port=5
  driveracc : Inport  Port=6
  curveunit : Inport  Port=7
  Add : Sum
  Add1 : Sum
  Constant1 : Constant  Value=0.2
  Divide : Product  Inputs=*/
  EndSpd : Scope
  Gain : Gain  Gain=3.6
  Inf : Constant  Value=inf  OutDataTypeStr=Inherit: Inherit via back propagation
  LearningCnt : Stateflow chart  TreatAsAtomicUnit=on
  LrnCnt : Scope  NumInputPorts=2
  Multiply : Gain  Gain=9.81
  NsafeUpdating : MATLAB Function  TreatAsAtomicUnit=on
  Product : Product
  Scope : Scope
  Square Root : Sqrt
  Switch : Switch  Criteria=u2 ~= 0  SaturateOnIntegerOverflow=off  InputSameDT=off
  Unit Delay : UnitDelay  SampleTime=-1  HasFrameUpgradeWarning=on
  Unit Delay1 : UnitDelay  SampleTime=-1  HasFrameUpgradeWarning=on
  final LrnCnt : Scope  NumInputPorts=2
  NsafeUpdate : Outport
  Out2 : Outport  Port=2
  Out3 : Outport  Port=3
  wires:
  LearningCnt/1(AccLrnCnt) -> Add/2, LrnCnt/1
  LearningCnt/2(BrkLrnCnt) -> Add1/1, LrnCnt/2
  CurrentRadius/1 -> LearningCnt/3(radius)
  accdmd/1 -> LearningCnt/4(accdmd)
  drvierbrk/1 -> LearningCnt/5(brk)
  driveracc/1 -> LearningCnt/6(acc)
  NsafeUpdating/1(y) -> NsafeUpdate/1
  VehicleSpd/1 -> LearningCnt/2(VehicleSpd)
  LearningCnt/3(EndSpd) -> Divide/1, Gain/1
  Constant1/1 -> Multiply/1
  Product/1 -> Square Root/1
  Square Root/1 -> Divide/2
  Divide/1 -> Out3/1, Scope/1  "Nsafe Reference"
  r_min/1 -> LearningCnt/1(r_min)
  Gain/1 -> Out2/1, EndSpd/1  "mps to kph"
  curveunit/1 -> LearningCnt/7(CurveUnit)
  Multiply/1 -> Product/2
  Inf/1 -> Switch/3
  LearningCnt/4(EndRadius) -> Switch/1, Switch/2
  Switch/1 -> Product/1
  [AccLrnCnt] -> NsafeUpdating/1(acc), final LrnCnt/1
  [BrkLrnCnt] -> NsafeUpdating/2(brk), final LrnCnt/2
  Add/1 -> [AccLrnCnt]
  Unit Delay/1 -> Add/1
  Add1/1 -> [BrkLrnCnt]
  Unit Delay1/1 -> Add1/2
  NsafeUpdating/3(newbrk) -> Unit Delay1/1
  NsafeUpdating/2(newacc) -> Unit Delay/1

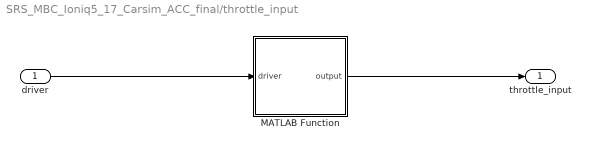
== system SRS_MBC_Ioniq5_17_Carsim_ACC_final/throttle_input ==
  driver : Inport
  MATLAB Function : MATLAB Function  TreatAsAtomicUnit=on
  throttle_input : Outport
  wires:
  driver/1 -> MATLAB Function/1(driver)
  MATLAB Function/1(output) -> throttle_input/1

== stateflow chart SRS_MBC_Ioniq5_17_Carsim_ACC_final/main chart ==
  state CurveRoadState
    en:
    v_init = vehicle_spd;
    v_final = srs_spd;
    dist = max_distance;
    [time_final_ori,  time_final_const, dist_const] = CalTimeUniformAccel(dist, v_init, v_final, a_min, t_margin);
    [a_1, a_2, a_3, a_4, a_5,a_min_ref] = MinJerkPolyCoef(v_init, v_final, dist, time_final_ori, a_min);
    disp(v_init);
    disp(v_final);
    disp(dist);
    disp(time_final_ori);
    if a_min_ref <= a_min
    [a_1, a_2, a_3, a_4, a_5, a_min_ref] = MinJerkPolyCoef(v_init, v_final, dist_const, time_final_const, a_min)
    time_final = time_final_const;
    distance = dist_const;
    else
    time_final=time_final_ori;
    distance = dist;
    end
  state InitialState
    en, du:
    a_1=0;
    a_2=0;
    a_3=0;
    a_4=0;
    a_5=0;
    time_final_ori = 0;
    driver = 0;
  state KeepSpdState
    driver = 0;
    time_final = 0;
    a_1=0;
    a_2=0;
    a_3=0;
    a_4=0;
    a_5=0;
  state NormAccelState_
    driver=1;
  state PowerAccelState
    driver=3;
  (default) -> InitialState
  InitialState -> CurveRoadState [order 2] : [curve_unit == 1 && vehicle_spd > srs_spd && radius ~= r_min]
  InitialState -> PowerAccelState [order 1] : [vehicle_spd == 0]
  (junction 185) -> InitialState : [after(1,tick)]
  InitialState -> (junction 181) [order 3] : [curve_unit == 0]
  CurveRoadState -> KeepSpdState : [vehicle_spd <= srs_spd || radius == r_min || driver_acc >= 0.01]
  (junction 171) -> (junction 185) : [radius > 2500]
  (junction 181) -> NormAccelState_
  KeepSpdState -> NormAccelState_ [order 1] : [curve_unit == 0 && radius > r_min]
  NormAccelState_ -> (junction 171)
  (junction 176) -> (junction 171)
  KeepSpdState -> (junction 176) [order 2]
  PowerAccelState -> (junction 176)
  data: dist function_input; time_final function_output; v_init function_input; v_final function_input; a_min function_input; t_margin function_input; time_final_const function_output; dist_const function_output; a_1 function_output; v_init function_input; v_final function_input; a_2 function_output; a_3 function_output; a_4 function_output; dist function_input; time_final function_input; a_min function_input; a_5 function_output; a_min_ref function_output; curve_unit input; r_min input; radius input; vehicle_spd input; srs_spd input; driver_acc input; a_1 output; a_2 output; a_3 output; a_4 output; a_5 output; driver output; time_final output; distance local; a_min input; t_margin input; max_distance input; v_init local; v_final local; time_final_ori local; time_final_const local; dist_const local; dist local; a_min_ref local
  function [time_final, time_final_const, dist_const] = CalTimeUniformAccel(dist, v_init, v_final, a_min, t_margin):
    | function [time_final, time_final_const, dist_const] = CalTimeUniformAccel(dist, v_init, v_final, a_min, t_margin)
    |     % radius: 입력 값
    |     % v0: 초기 속도
    |     % vf: 최종 속도
    |     % dist: 최속 곡률 반지름까지 남은 거리
    |     % tf: 계산된 시간 (dist / ((v0 + vf) / 2))
    |     
    |     % tf 계산 (dist NaN이 아니면 계산)
    |     if ~isnan(dist)
    |         time_final = dist / ((v_init + v_final) / 2);  % 평균 속도를 사용하여 시간 계산
    |     else
    |         time_final = NaN;  % distance가 유효하지 않으면 tf도 NaN으로 설정
    |     end
    | 
    |     %% constraint 고려했을 때
    | 
    |     % -3 < 3(vf - v0)/(2*tf) 를 만족하는 최소 tf 계산
    |     numerator = 3 * (v_final - v_init);
    |     denominator = 2 * a_min;
    | 
    |     % 계산된 tf 경계값
    |     tf_candidate = numerator / denominator;
    | 
    |     %tf는 양수여야 하므로 0보다 작으면 무의미
    |     if tf_candidate <= 0
    |         time_final_const = NaN;  % 또는 예외 처리
    |         dist_const = NaN;
    |         return;
    |     end
    | 
    |     % replanning tf_const 계산
    |     time_final_const = ceil(tf_candidate * 10) / 10 + t_margin;
    |     dist_const = time_final_const * (v_init + v_final) / 2;
  function [a_1, a_2, a_3, a_4, a_5, a_min_ref] =  MinJerkPolyCoef(v_init, v_final, dist, time_final, a_min):
    | function [a_1, a_2, a_3, a_4, a_5, a_min_ref] =  MinJerkPolyCoef(v_init, v_final, dist, time_final, a_min)
    | 
    | %% 5차 profiling %%
    | x0 = 0;
    | xf = dist;
    | tf = time_final;
    | a0 = 0;
    | af = 0; %임의로 지정
    | v0 = v_init;
    | vf = v_final;
    | 
    | P = [1, 0, 0, 0, 0, 0;
    |     0, 1, 0, 0, 0, 0;
    |     0, 0, 2, 0, 0, 0; 
    |     1, tf, tf^2, tf^3, tf^4, tf^5;
    |     0, 1, 2*tf, 3*tf^2, 4*tf^3, 5*tf^4;
    |     0, 0, 2, 6*tf, 12*tf^2, 20*tf^3;];
    | 
    | Q = [x0; v0; a0; xf; vf; af;];
    | 
    | % 연립 방정식 풀기 (A \ B 사용)
    | coeffs = P \ Q;
    | 
    | % 계수 추출
    | a_1 = coeffs(2);
    | a_2 = coeffs(3);
    | a_3 = coeffs(4);
    | a_4 = coeffs(5);
    | a_5 = coeffs(6);
    | 
    | %% solve Jerk Root: j(t) = 6*b3 + 24*b4*t + 60*b5*t^2 = 0 의 해 계산 %%
    | % 입력: a3, a4, a5
    | % 출력: t1, t2 (두 개의 실근 또는 복소수근 반환)
    | 
    | % 계수 설정 (표준 2차형식 At^2 + Bt + C)
    | A = 60 * a_5;
    | B = 24 * a_4;
    | C = 6  * a_3;
    | 
    | % 판별식 계산
    | D = B^2 - 4*A*C;
    | 
    | % 해 계산
    | if A == 0
    | % 선형 방정식으로 처리 (예외 처리)
    |     if B ~= 0
    |         t1 = -C / B;
    |         t2 = NaN;  % 두 번째 해 없음
    |     else
    |         t1 = NaN;
    |         t2 = NaN;
    |     end
    | else
    |     sqrtD = sqrt(D);  % D < 0이면 복소수 처리됨
    |     t1 = (-B - sqrtD) / (2*A);
    |     t2 = (-B + sqrtD) / (2*A);
    | end
    | % minAcceleration: 두 시간점에서의 가속도를 계산해 더 작은 값 반환
    | 
    | % 각 시간점에서의 가속도 계산
    | a_t1 = 2 * a_2 + 6 * a_3 * t1 + 12 * a_4 * t1^2 + 20 * a_5 * t1^3;
    | a_t2 = 2 * a_2 + 6 * a_3 * t2 + 12 * a_4 * t2^2 + 20 * a_5 * t2^3;
    | 
    | % 둘 다 유효한 숫자인 경우
    | if ~isnan(a_t1) && ~isnan(a_t2)
    |     a_min_ref = min(a_t1, a_t2);
    | 
    | % 하나만 유효한 경우
    | elseif ~isnan(a_t1)
    |     a_min_ref = a_t1;
    | elseif ~isnan(a_t2)
    |     a_min_ref = a_t2;
    | 
    | % 둘 다 유효하지 않은 경우
    | else
    |     a_min_ref = NaN;
    | end
    | %% 임계값을 넘어가면 constraint를 고려하여 계수 재계산 및 확정 %%
    | if a_min_ref <= a_min
    |    a_1 = 0;
    |    a_2 = 0;
    |    a_3 = 0;
    |    a_4 = 0;
    |    a_5 = 0;
    | end

== stateflow chart SRS_MBC_Ioniq5_17_Carsim_ACC_final/aggressive driver model/Chart ==
  state INITIAL
    driveracc = 0;
    driverbrk = 0;
  state AccelOn
    driveracc = 1;
  state BrkOn
    driverbrk = 1;
  (default) -> INITIAL
  INITIAL -> AccelOn [order 1] : [r_min > 0 && radius <= 150 && desspd > 0 && desspd > spd + 0.5]
  AccelOn -> INITIAL : [(desspd < spd+0.25 && desspd > spd -0.25) || r_min == 0]
  BrkOn -> INITIAL : [(desspd < spd+0.25 && desspd > spd -0.25) || r_min == 0]
  INITIAL -> BrkOn [order 2] : [r_min > 0 && radius <= 150 && desspd > 0 && desspd < spd - 0.5]
  data: desspd input; r_min input; driveracc output; spd input; radius input; driverbrk output

== matlab function SRS_MBC_Ioniq5_17_Carsim_ACC_final/MATLAB Function1 ==
  data: time input; t_output output; time_final input; p output
function [t_output, p] = fcn(time, time_final)
    persistent prev_time;  % 이전 시간 저장용 변수
    if isempty(prev_time)
        prev_time = time;  % 초기화, 첫 호출 시 현재 시간으로 설정
    end

    % time이 time_final에 도달하면 prev_time을 초기화
    if (time - prev_time) < time_final 
        t_output = (time - prev_time);  % time_final에 도달하기 전까지의 값
        p = prev_time;

    
    elseif (time - prev_time) == time_final 
        t_output = 0;  % time_final에 도달하기 전까지의 값
        p = prev_time;

    else
        prev_time = time;  % 새로운 loop 시작 (time_final 도달 후 초기화)
        t_output = 0;  % time_final 도달 후 초기화된 slow_time
        p = prev_time;

    end

end

== matlab function SRS_MBC_Ioniq5_17_Carsim_ACC_final/throttle_input/MATLAB Function ==
  data: driver input; output output
function output = driver_function(driver)
    switch driver
        case 0
            output = 0;
        case 1
            output = 0.1;
        case 2
            output = 0.02;
        otherwise
            output = 0.2;
    end
end

== stateflow chart SRS_MBC_Ioniq5_17_Carsim_ACC_final/RminStore ==
  state RminStopStoring
    Rmin = minimum;
    RminStart = 0;
  state RminStoring
    if r>2500 && r<3000
    minimum = r-2500;
    end
    Rmin = minimum;
    RminStart = minimum;
  state INITIAL
    minimum = 0;
    Rmin=0;
    RminStart=0;
  (default) -> INITIAL
  INITIAL -> RminStoring : [r > 2500 && r < 3000]
  RminStoring -> RminStopStoring : [minimum == r]
  (junction 14) -> INITIAL
  RminStopStoring -> (junction 14) : [minimum < r]
  data: r input; Rmin output; minimum local; RminStart output

== matlab function SRS_MBC_Ioniq5_17_Carsim_ACC_final/MATLAB Function ==
  data: u input; y output
function y = fcn(u)

if u <= 475.5
    y = 475.5-u;
elseif u <= 1217
        y = 1217-u;
elseif u <= 1958.5
        y = 1958.5-u;
elseif u <= 2700
        y = 2700-u;
else
    y=0;
end

== stateflow chart SRS_MBC_Ioniq5_17_Carsim_ACC_final/learning algorithm/LearningCnt ==
  state BrkLrnEna
    en:
    EnaSta = 1;
    curveEnter = 0;
    ex:
    if BrkLrnSta == 0;
    BrkLrnSta = 1;
    else
    BrkLrnSta = BrkLrnSta + 1;
    end
  state DriverBrk
    en:
    curveEnter = 1;
  state SaveEndSpd
    ex:
    SaveSpd = VehicleSpd;
    SaveRadius = radius;
    EnaSta = 0;
    % 개입 끝날 때의 속도 저장
  state SRSMBC
    %BrkPedal=StrkDpthPcVal;
    %AccPdeal=AccPedDepVal;
    EndSpd = 0;
  state INIT
    BrkLrnSta = 0;
    AccLrnSta = 0;
    curveEnter = 0;
    SaveSpd = 0;
    SaveRadius = 0;
    EndSpd = 0;
  state CurveOut
    en:
    if (BrkLrnSta ~= 0 && AccLrnSta~= 0)
    %acc, brk 번갈아 개입
    BrkLrnCnt = 0;
    AccLrnCnt = 0;
    EndSpd = 0;
    disp(AccLrnSta);
    elseif (BrkLrnSta > 0 && AccLrnSta == 0)
    BrkLrnCnt = 1;
    EndSpd = SaveSpd;
    EndRadius = SaveRadius;
    %brk만 개입
    elseif (BrkLrnSta == 0 && AccLrnSta > 0)
    AccLrnCnt = 1;
    EndSpd = SaveSpd;
    EndRadius = SaveRadius;
    %acc만 개입
    end
    EndSpd = SaveSpd;
    ex:
    BrkLrnCnt = 0;
    AccLrnCnt = 0;
  state DriverAcc
    en:
    curveEnter = 1;
  state AccLrnEna
    en:
    EnaSta = 1;
    curveEnter = 0;
    ex:
    if AccLrnSta == 0;
    AccLrnSta = 1;
    else
    AccLrnSta = AccLrnSta +1;
    end
  (junction 163) -> (junction 165)
  BrkLrnEna -> (junction 163) [order 1] : [brk <= 8.5]
  (junction 165) -> SaveEndSpd
  BrkLrnEna -> (junction 250) [order 2] : [(acc == 0 && brk == 0 && radius == r_min) || CurveUnit == 0]
  (junction 250) -> CurveOut
  DriverBrk -> BrkLrnEna [order 2] : [brk > 8.5]
  DriverBrk -> (junction 273) [order 1] : [(acc <= 0.05 && brk <= 0.05 && radius == r_min) || CurveUnit == 0]
  (junction 273) -> CurveOut
  DriverBrk -> SRSMBC [order 3] : [brk <= 0.05]
  SRSMBC -> DriverBrk [order 1] : [brk>0.05]
  (default) -> INIT
  SaveEndSpd -> (junction 240) [order 1] : [CurveUnit == 0]
      | % 운전자 개입 off
  (junction 240) -> CurveOut
  SaveEndSpd -> SRSMBC [order 2] : [brk <= 0.05 && acc <= 0.05 && CurveUnit == 1]
  INIT -> SRSMBC : [CurveUnit == 1 && accdmd < -0.01 && radius > r_min]
      | % 곡률 진입 중일 때만 SRS_MBC 필요
  (junction 270) -> INIT
  DriverAcc -> SRSMBC [order 3] : [acc <=0.05]
  SRSMBC -> DriverAcc [order 2] : [acc>0.05]
  SRSMBC -> (junction 237) [order 3] : [(acc == 0 && brk == 0 && radius == r_min) || CurveUnit == 0]
  (junction 178) -> SaveEndSpd
  (junction 279) -> SaveEndSpd
  (junction 237) -> CurveOut
  DriverAcc -> (junction 279) [order 1] : [acc <= 0.05 && brk <= 0.05]
  DriverAcc -> AccLrnEna [order 2] : [acc>6.5]
  (junction 245) -> CurveOut
  CurveOut -> (junction 268) : [after(1,tick)]
  AccLrnEna -> (junction 245) [order 1] : [(acc == 0 && brk == 0 && radius == r_min) || CurveUnit == 0]
  AccLrnEna -> (junction 176) [order 2] : [acc <= 6.5]
  (junction 176) -> (junction 178)
  (junction 268) -> (junction 270)
  data: r_min input; VehicleSpd input; AccLrnCnt output; BrkLrnCnt output; radius input; accdmd input; brk input; acc input; EndSpd output; EnaSta local; curveEnter local; CurveUnit input; BrkLrnSta local; AccLrnSta local; SaveSpd local; SaveRadius local; EndRadius output

== matlab function SRS_MBC_Ioniq5_17_Carsim_ACC_final/learning algorithm/NsafeUpdating ==
  data: acc input; y output; newacc output; newbrk output; brk input
function [y,newacc,newbrk] = fcn(acc, brk)

if acc > brk && acc == 2
    y = 0.1; % nsafe 증가
    newacc = 0;
    newbrk = 0; % 학습 값 초기화
elseif brk > acc && brk == 2
    y = -0.1; % nsafe 감소
    newacc = 0;
    newbrk = 0; % 학습 값 초기화
else
    y = 0; % nsafe 유지
    newacc = acc;
    newbrk = brk; % 현재 값 상속
end
